simulink model "camera_comm"  (R2018a)
settings: Solver=FixedStepAuto  StartTime=0.0  StopTime=inf  RelTol=1e-3  EnableMultiTasking=on
libraries: embdlinuxlib x4, simulink x4, dspstat3 x2
settings Model: SimulationMode=external  Creator=Martin  LastModifiedBy=Lenovo
settings SolverCC: PositivePriorityOrder=on
settings OptimizationCC: EnhancedBackFolding=on  PassReuseOutputArgsAs=Individual arguments  MaxStackSize=64  OptimizeBlockOrder=speed  DifferentSizesBufferReuse=on  OptimizationCustomize=off
settings DebuggingCC: ParameterTunabilityLossMsg=error
settings HardwareCC: ProdBitPerPointer=32  ProdBitPerSizeT=32  ProdBitPerPtrDiffT=32  ProdLargestAtomicInteger=Long  ProdLargestAtomicFloat=Double  ProdWordSize=32  ProdHWDeviceType=ARM Compatible->ARM Cortex
settings SFSimCC: MATLABDynamicMemAlloc=off
settings RTWCC: SystemTargetFile=ert.tlc  HardwareBoard=Raspberry Pi  TLCOptions="-aInlineSetEventsForThisBaseRateFcn=TLC_FALSE -aSuppressMultiTaskScheduler=TLC_FALSE  -aRateBasedStepFcn=0"  TemplateMakefile=ert_default_tmf  GenerateReport=on  Toolchain=GNU GCC Raspberry Pi  BuildConfiguration=Faster Runs  IncludeHyperlinkInReport=on  LaunchReport=on  GenerateTraceInfo=on  GenerateTraceReport=on  GenerateTraceReportSl=on  GenerateTraceReportSf=on  GenerateTraceReportEml=on
settings CodeAppCC: ForceParamTrailComments=on  IgnoreCustomStorageClasses=off  OperatorAnnotations=on  SimulinkDataObjDesc=on  SFDataObjDesc=on  InsertBlockDesc=on
settings ERTTargetCC: SupportVariableSizeSignals=on

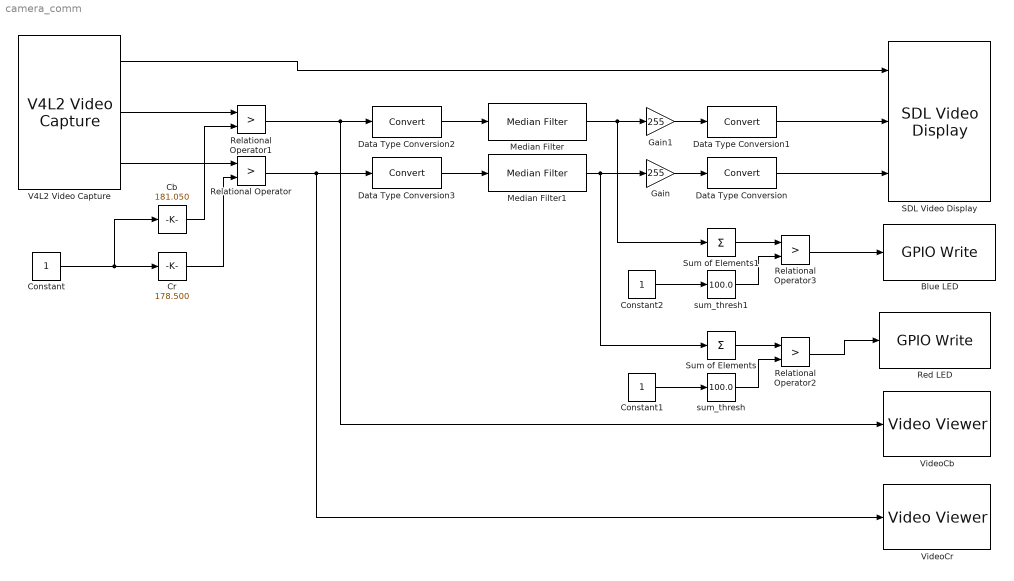
== system camera_comm ==
  Blue LED : embdlinuxlib/GPIO Write  board=Pi 2 Model B  gpio=24  direction=Output  blockPlatform=Raspberry Pi
      settings: SourceProductName=Simulink Support Package for Raspberry Pi Hardware  SourceProductBaseCode=RASPPI
  Cb : simulink/Math Operations/Slider Gain  gain=181.050  low=0  high=255
  Constant : Constant
  Constant1 : Constant
  Constant2 : Constant
  Cr : simulink/Math Operations/Slider Gain  gain=178.500  low=0  high=255
  Data Type Conversion{,1..3} (4 alike) : DataTypeConversion
  Gain : Gain  Gain=255
  Gain1 : Gain  Gain=255
  Median Filter : dspstat3/Median Filter  WindowLength=5  SimulateUsing=Interpreted execution
      settings: SourceProductName=DSP System Toolbox  SourceProductBaseCode=DS
  Median Filter1 : dspstat3/Median Filter  WindowLength=5  SimulateUsing=Interpreted execution
      settings: SourceProductName=DSP System Toolbox  SourceProductBaseCode=DS
  Red LED : embdlinuxlib/GPIO Write  board=Pi 2 Model B  gpio=23  direction=Output  blockPlatform=Raspberry Pi
      settings: SourceProductName=Simulink Support Package for Raspberry Pi Hardware  SourceProductBaseCode=RASPPI
  Relational Operator{,1..3} (4 alike) : RelationalOperator  Operator=>  OutDataTypeStr=boolean  RndMeth=Simplest
  SDL Video Display : embdlinuxlib/SDL Video Display  pixelFormat=YCbCr 4:2:2  pixelOrder=Planar  rowMajor=on  blockPlatform=Raspberry Pi
      settings: SourceProductName=Simulink Support Package for Raspberry Pi Hardware  SourceProductBaseCode=RASPPI
  Sum of Elements : Sum  Inputs=+
  Sum of Elements1 : Sum  Inputs=+
  V4L2 Video Capture : embdlinuxlib/V4L2 Video Capture  m_devName='/dev/video0'  roi=[0, 0, 640, 480]  imSizeSelection=160x120  imSize=[640, 480]  pixelFormat=YCbCr 4:2:2  pixelOrder=Planar  sampleTime=1/10  simOutput=Colorbars  blockPlatform=Raspberry Pi
      settings: SourceProductName=Simulink Support Package for Raspberry Pi Hardware  SourceProductBaseCode=RASPPI
  VideoCb : VideoViewer  FigPos=[1344 783 418 304]
  "VideoCr " : VideoViewer  FigPos=[1344 783 418 304]
  sum_thresh : simulink/Math Operations/Slider Gain  gain=100.0  low=0  high=1000
  sum_thresh1 : simulink/Math Operations/Slider Gain  gain=100.0  low=0  high=1000
  wires:
  V4L2 Video Capture/1 -> SDL Video Display/1
  V4L2 Video Capture/3 -> Relational Operator/1
  Constant/1 -> Cb/1, Cr/1
  Cr/1 -> Relational Operator/2
  Relational Operator/1 -> Data Type Conversion3/1, "VideoCr "/1
  Data Type Conversion/1 -> SDL Video Display/3
  Gain/1 -> Data Type Conversion/1
  Gain1/1 -> Data Type Conversion1/1
  Data Type Conversion1/1 -> SDL Video Display/2
  Relational Operator1/1 -> Data Type Conversion2/1, VideoCb/1
  V4L2 Video Capture/2 -> Relational Operator1/1
  Cb/1 -> Relational Operator1/2
  Sum of Elements/1 -> Relational Operator2/1
  Constant1/1 -> sum_thresh/1
  sum_thresh/1 -> Relational Operator2/2
  Relational Operator2/1 -> Red LED/1
  Median Filter/1 -> Sum of Elements1/1, Gain1/1
  Median Filter1/1 -> Gain/1, Sum of Elements/1
  Relational Operator3/1 -> Blue LED/1
  sum_thresh1/1 -> Relational Operator3/2
  Constant2/1 -> sum_thresh1/1
  Sum of Elements1/1 -> Relational Operator3/1
  Data Type Conversion2/1 -> Median Filter/1
  Data Type Conversion3/1 -> Median Filter1/1
